simulink model "loop_filters"  (Simulink 6.6)
settings: Solver=VariableStepDiscrete  StartTime=0.0  StopTime=10  RelTol=1e-3
PreLoadFcn:
  | Fs = 1000;
StopFcn:
  | doFFTplot(Fs, [LoopFilter1,LoopFilter2], ['Loop Filter 1';'Loop Filter 2'], 1, 4, 'hann');
libraries: xbsIndex_r4 x10, dspsrcs4 x1
settings Model: Creator=lcrockett  LastModifiedBy=lcrockett

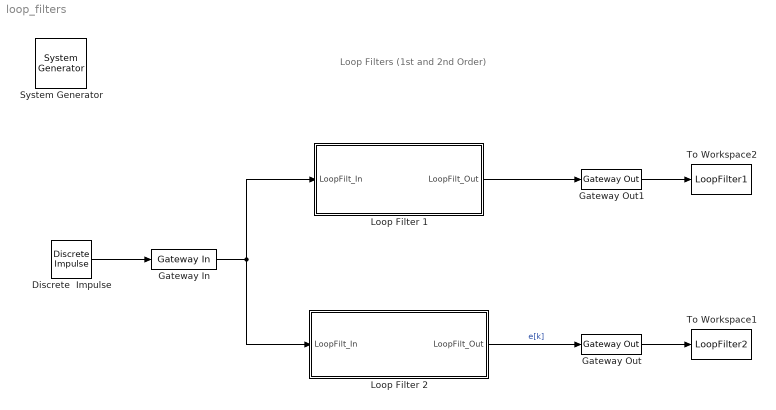
== system loop_filters ==
  note: Loop Filters (1st and 2nd Order)
  " System Generator" : xbsIndex_r4/ System Generator  Tag=genX  SystemSampleTime=-1  xilinxfamily=virtex4  part=xc4vsx35  speed=-10  package=ff668  synthesis_tool=XST  clock_wrapper=Clock Enables  directory=./netlist  testbench=off  simulink_period=1/Fs  sysclk_period=10  dcm_input_clock_period=100  incr_netlist=off  trim_vbits=Everywhere in SubSystem  dbl_ovrd=According to Block Masks  core_generation=According to Block Masks  run_coregen=off  deprecated_control=off  eval_field=0  block_type=sysgen
      settings: block_version=9.2.01
  Discrete  Impulse : dspsrcs4/Discrete  Impulse  Delay=0  SampleTime=1  FrameSample=1  dataType=double  isSigned=on  wordLen=16  udDataType=sfix(16)  fracBitsMode=Best precision  numFracBits=15
  Gateway In : xbsIndex_r4/Gateway In  arith_type="Signed  (2's comp)"  n_bits=32  bin_pt=30  quantization="Round  (unbiased: +/- Inf)"  overflow=Saturate  period=1/Fs  dbl_ovrd=off  timing_constraint=None  locs_specified=off  LOCs={}  block_type=gatewayin
      settings: infoedit="Gateway in block.  Converts inputs of type Simulink integer, double and fixed point to  Xilinx fixed point type.<P><P>Hardware notes:  In hardware these blocks become top level input ports."  block_version=9.2.01
  Gateway Out : xbsIndex_r4/Gateway Out  hdl_port=on  timing_constraint=None  locs_specified=off  LOCs={}  block_type=gatewayout
      settings: infoedit="Gateway out block.  Converts Xilinx fixed point inputs into ouputs of type Simulink integer, double, or fixed point.<P><P>Hardware notes:  In hardware these blocks become top level output ports or are discarded, depending on how they are configured."  block_version=9.2.01
  Gateway Out1 : xbsIndex_r4/Gateway Out  hdl_port=on  timing_constraint=None  locs_specified=off  LOCs={}  block_type=gatewayout
      settings: infoedit="Gateway out block.  Converts Xilinx fixed point inputs into ouputs of type Simulink integer, double, or fixed point.<P><P>Hardware notes:  In hardware these blocks become top level output ports or are discarded, depending on how they are configured."  block_version=9.2.01
  Loop Filter 1 : Subsystem  mask(Loop Filter Parameters){alpha_n=3, phase_det_word=32}
      mask prompts: alpha_n "Alpha (bits to shift right by)"; phase_det_word "Input wordlength"
      mask help: The first order loop filter contains a proportional path only, with coefficient Alpha. This constant multiplication is implemented as a shift.
      mask init:
      | alpha_shift_wl = phase_det_word + alpha_n;
  Loop Filter 2 : Subsystem  mask(Loop Filter Parameters){alpha_n=3, beta_n=7, phase_det_word=32, acc_ibits=10}
      mask prompts: alpha_n "Alpha (bits to shift right by)"; beta_n "Beta (bits to shift right by)"; phase_det_word "Input wordlength"; acc_ibits "Accumulator integer bits"
      mask help:
      | The loop filter contains two paths: a proportional path and an integral path. These have coefficients Alpha, and [Alpha x Beta], respectively.
      |
      | The wordlengths at the outputs of the shifts are extended by the degrees of the shifts. This also defines the number of fractional bits required in the accumulator of the integrator. The number of whole bits should be sufficient to prevent overflow.
      mask init:
      | alpha_shift_wl = phase_det_word + alpha_n;
      | beta_shift_wl = phase_det_word + beta_n;
  To Workspace1 : ToWorkspace  VariableName=LoopFilter2  SampleTime=-1  SaveFormat=Array
  To Workspace2 : ToWorkspace  VariableName=LoopFilter1  SampleTime=-1  SaveFormat=Array
  wires:
  Loop Filter 2/1(LoopFilt_Out) -> Gateway Out/1  "e[k]"
  Discrete  Impulse/1 -> Gateway In/1
  Gateway In/1 -> Loop Filter 2/1(LoopFilt_In), Loop Filter 1/1(LoopFilt_In)
  Gateway Out/1 -> To Workspace1/1
  Loop Filter 1/1(LoopFilt_Out) -> Gateway Out1/1
  Gateway Out1/1 -> To Workspace2/1

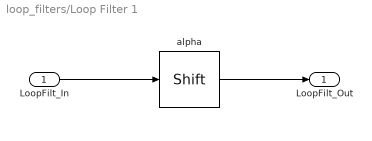
== system loop_filters/Loop Filter 1 ==
  LoopFilt_In : Inport
  alpha : xbsIndex_r4/Shift  shift_dir=Right  shift_bits=alpha_n  en=off  latency=0  precision=User Defined  arith_type="Signed  (2's comp)"  n_bits=alpha_shift_wl  bin_pt=alpha_shift_wl-2  quantization=Truncate  overflow=Wrap  dbl_ovrd=off  block_type=shift
      settings: block_version=9.2.01
  LoopFilt_Out : Outport
  wires:
  alpha/1 -> LoopFilt_Out/1
  LoopFilt_In/1 -> alpha/1

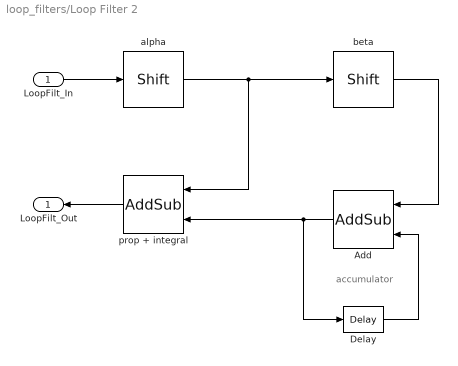
== system loop_filters/Loop Filter 2 ==
  note: accumulator
  LoopFilt_In : Inport
  Add : xbsIndex_r4/AddSub  Orientation=left  mode=Addition  use_carryin=off  use_carryout=off  en=off  latency=0  precision=User Defined  arith_type="Signed  (2's comp)"  n_bits=acc_ibits+beta_shift_wl-2  bin_pt=beta_shift_wl-2  quantization="Round  (unbiased: +/- Inf)"  overflow=Wrap  dbl_ovrd=off  use_behavioral_HDL=off  pipelined=off  use_rpm=on  block_type=addsub
      settings: block_version=9.2.01
  Delay : xbsIndex_r4/Delay  en=off  latency=1  dbl_ovrd=off  reg_retiming=off  block_type=delay
      settings: block_version=9.2.01
  alpha : xbsIndex_r4/Shift  shift_dir=Right  shift_bits=alpha_n  en=off  latency=0  precision=User Defined  arith_type="Signed  (2's comp)"  n_bits=alpha_shift_wl  bin_pt=alpha_shift_wl-2  quantization=Truncate  overflow=Wrap  dbl_ovrd=off  block_type=shift
      settings: block_version=9.2.01
  beta : xbsIndex_r4/Shift  shift_dir=Right  shift_bits=beta_n  en=off  latency=0  precision=User Defined  arith_type="Signed  (2's comp)"  n_bits=beta_shift_wl  bin_pt=beta_shift_wl-2  quantization=Truncate  overflow=Wrap  dbl_ovrd=off  block_type=shift
      settings: block_version=9.2.01
  prop + integral : xbsIndex_r4/AddSub  Orientation=left  mode=Addition  use_carryin=off  use_carryout=off  en=off  latency=0  precision=Full  arith_type="Signed  (2's comp)"  n_bits=20  bin_pt=14  quantization="Round  (unbiased: +/- Inf)"  overflow=Wrap  dbl_ovrd=off  use_behavioral_HDL=off  pipelined=off  use_rpm=on  block_type=addsub
      settings: block_version=9.2.01
  LoopFilt_Out : Outport  Orientation=left
  wires:
  Add/1 -> Delay/1, prop + integral/2
  Delay/1 -> Add/2
  LoopFilt_In/1 -> alpha/1
  prop + integral/1 -> LoopFilt_Out/1
  alpha/1 -> prop + integral/1, beta/1
  beta/1 -> Add/1
